simulink model "model"  (R2016a)
settings: Solver=VariableStepAuto  StartTime=0.0  StopTime=100  RelTol=1e-3
settings Model: Creator=Florian  LastModifiedBy=Florian

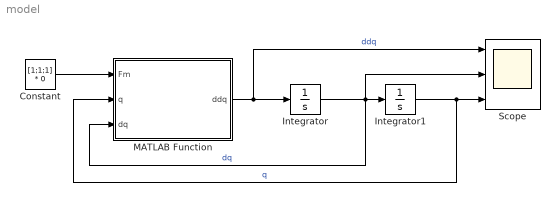
== system model ==
  Constant : Constant  Value=[1;1;1] * 0
  Integrator : Integrator  InitialCondition=[0;0;0]
  Integrator1 : Integrator  InitialCondition=[0.14; 0.14; 0.14]
  MATLAB Function : MATLAB Function  TreatAsAtomicUnit=on
  Scope : Scope  NumInputPorts=3
  wires:
  MATLAB Function/1(ddq) -> Scope/1, Integrator/1  "ddq"
  Integrator/1 -> Scope/2, MATLAB Function/3(dq), Integrator1/1  "dq"
  Integrator1/1 -> Scope/3, MATLAB Function/2(q)  "q"
  Constant/1 -> MATLAB Function/1(Fm)

== matlab function model/MATLAB Function ==
  data: Fm input; ddq output; q input; dq input
function ddq = fcn(Fm, q, dq)
%#codegen

coder.extrinsic('Mfunc');
coder.extrinsic('Nfunc');

if abs(q(1) - q(2)) < 0.0001 && abs(q(2) - q(3)) < 0.0001
    M = Mfunc2(q);
    N = Nfunc2(q, dq);
    Q = Qfunc2(dq, Fm);    
else
    M = Mfunc(q);
    N = Nfunc(q, dq);
    Q = Qfunc(dq, Fm);  
end

invM = inv(M);
ddq = invM * (-Q + N);
if abs(q(1) - 0.16) < 0.001
    help = 1+1;
end
